simulink model "CLIK_II_ORDINE"  (R2019b)
settings: Solver=VariableStepAuto  StartTime=0.0  StopTime=T(end)  RelTol=1e-3
undefined symbols (not defined in the file): a1, a2, d0, DiscIntNeverNeededParam, q0
settings Model: Creator=damia  LastModifiedBy=Alessandro
settings DataIOCC: ReturnWorkspaceOutputs=off
settings DebuggingCC: ArithmeticOperatorsInVariantConditions=warning
settings SFSimCC: CustomCodeUndefinedFunction=UseInterfaceOnly

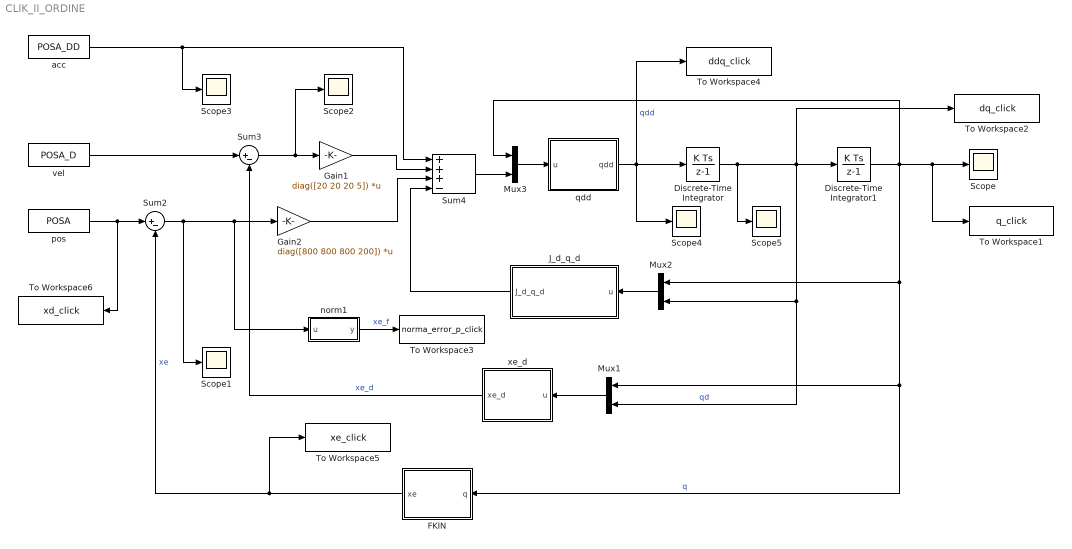
== system CLIK_II_ORDINE ==
  Discrete-Time Integrator : DiscreteIntegrator  InitialCondition=zeros(1,4)  SampleTime=1e-3  ICPrevOutput=DiscIntNeverNeededParam  ICPrevScaledInput=DiscIntNeverNeededParam
  Discrete-Time Integrator1 : DiscreteIntegrator  InitialCondition=q0  SampleTime=1e-3  ICPrevOutput=DiscIntNeverNeededParam  ICPrevScaledInput=DiscIntNeverNeededParam
  FKIN : MATLAB Function  TreatAsAtomicUnit=on
  Gain1 : Gain  Gain=diag([20 20 20 5])  Multiplication=Matrix(K*u)
  Gain2 : Gain  Gain=diag([800 800 800 200])  Multiplication=Matrix(K*u)
  J_d_q_d : MATLAB Function  TreatAsAtomicUnit=on
  Mux1 : Mux  Inputs=2
  Mux2 : Mux  Inputs=2
  Mux3 : Mux  Inputs=2
  Scope{,1..5} (6 alike) : Scope
  Sum2 : Sum  Inputs=|+-
  Sum3 : Sum  Inputs=|+-
  Sum4 : Sum  Inputs=+++-
  To Workspace1 : ToWorkspace  VariableName=q_click  SaveFormat=Timeseries  SampleTime=-1
  To Workspace2 : ToWorkspace  VariableName=dq_click  SaveFormat=Timeseries  SampleTime=-1
  To Workspace3 : ToWorkspace  VariableName=norma_error_p_click  SaveFormat=Timeseries  SampleTime=-1
  To Workspace4 : ToWorkspace  VariableName=ddq_click  SaveFormat=Timeseries  SampleTime=-1
  To Workspace5 : ToWorkspace  VariableName=xe_click  SaveFormat=Timeseries  SampleTime=-1
  To Workspace6 : ToWorkspace  VariableName=xd_click  SaveFormat=Timeseries  SampleTime=-1
  acc : FromWorkspace  VariableName=POSA_DD  SampleTime=0.001
  norm1 : MATLAB Function  TreatAsAtomicUnit=on
  "pos " : FromWorkspace  VariableName=POSA  SampleTime=0.001
  qdd : MATLAB Function  TreatAsAtomicUnit=on
  "vel " : FromWorkspace  VariableName=POSA_D  SampleTime=0.001
  xe_d : MATLAB Function  TreatAsAtomicUnit=on
  wires:
  "pos "/1 -> Sum2/1, To Workspace6/1
  "vel "/1 -> Sum3/1
  Sum3/1 -> Scope2/1, Gain1/1
  Sum2/1 -> norm1/1(u), Gain2/1, Scope1/1
  Gain1/1 -> Sum4/2
  Gain2/1 -> Sum4/3
  acc/1 -> Scope3/1, Sum4/1
  Sum4/1 -> Mux3/2
  qdd/1(qdd) -> To Workspace4/1, Discrete-Time Integrator/1, Scope4/1  "qdd"
  Discrete-Time Integrator/1 -> Scope5/1, To Workspace2/1, Mux2/2, Mux1/2, Discrete-Time Integrator1/1  "qd"
  Discrete-Time Integrator1/1 -> To Workspace1/1, Scope/1, Mux3/1, Mux2/1, Mux1/1, FKIN/1(q)  "q"
  FKIN/1(xe) -> To Workspace5/1, Sum2/2  "xe"
  Mux3/1 -> qdd/1(u)
  xe_d/1(xe_d) -> Sum3/2  "xe_d"
  Mux1/1 -> xe_d/1(u)
  Mux2/1 -> J_d_q_d/1(u)
  J_d_q_d/1(J_d_q_d) -> Sum4/4
  norm1/1(y) -> To Workspace3/1  "xe_f"

== matlab function CLIK_II_ORDINE/xe_d ==
  data: u input; xe_d output; a1 parameter; a2 parameter
function xe_d = fcn(u, a1, a2)

q = u(1:4);
u2 = u(5:8);

% Jacobiano
J = [ -a1*sin(q(1))-a2*sin(q(1)+q(2))   -a2*sin(q(1)+q(2))  0   0   ;
       a1*cos(q(1))+a2*cos(q(1)+q(2))    a2*cos(q(1)+q(2))  0   0   ;
                   0                              0         1   0   ;
                   1                              1         0   1   ];
               
    xe_d = J*u2;
end

== matlab function CLIK_II_ORDINE/FKIN ==
  data: q input; xe output; a2 parameter; a1 parameter; d0 parameter
function xe = fcn(q, a2, a1, d0)

theta1 = q(1);
theta2 = q(2);
d3 = q(3);
theta4 = q(4);

% Cinematica diretta
xe = [a1*cos(theta1)+a2*cos(theta1+theta2) ;
      a1*sin(theta1)+a2*sin(theta1+theta2) ;
      d3+d0 ;
      theta1+theta2+theta4; ];
end

== matlab function CLIK_II_ORDINE/qdd ==
  data: u input; qdd output; a1 parameter; a2 parameter
function qdd = fcn(u, a1, a2)

q = u(1:4);
u2 = u(5:8);

% Jacobiano
J = [ -a1*sin(q(1))-a2*sin(q(1)+q(2))   -a2*sin(q(1)+q(2))  0   0   ;
       a1*cos(q(1))+a2*cos(q(1)+q(2))    a2*cos(q(1)+q(2))  0   0   ;
                   0                              0         1   0   ;
                   1                              1         0   1   ];

% Damped Least Squares
intervallo = 0.05;
k = 0.1;

if(abs(det(J))) < intervallo;
    J = J' * inv(J*J' + eye(4)*k^2);
    qdd = J*(u2);
else
    qdd = inv(J)*(u2);
end

== matlab function CLIK_II_ORDINE/J_d_q_d ==
  data: u input; J_d_q_d output; a1 parameter; a2 parameter
function J_d_q_d = fcn(u, a1, a2)

q = u(1:4);
q1_d=u(5);
q2_d=u(6);
u2 = u(5:8);
% Jacobiano derivato
               
J_d = [ (-q1_d + q2_d)*(a2*cos(q(1)+q(2)))-q1_d*a1*cos(q(1)),  -(q1_d+q2_d)*(a2*cos(q(1)+q(2))),   0,  0;
         -(q1_d+q2_d)*(a2*sin(q(1)+q(2)))-q1_d*a1*sin(q(1)),  -(q1_d+q2_d)*(a2*sin(q(1)+q(2))),   0,  0;
         0, 0, 0, 0;
         0, 0, 0, 0;];
               
J_d_q_d = J_d*u2;
    
end

== matlab function CLIK_II_ORDINE/norm1 ==
  data: u input; y output
function y = norm(u)
y = norm(u);
